simulink model "Problem3_ThreePhase_Inverter"  (R2025b)
settings: Solver=ode23t  StartTime=0.0  StopTime=0.1  MaxStep=1e-5  RelTol=1e-3
settings Model: Creator=Rashid  LastModifiedBy=Rashid

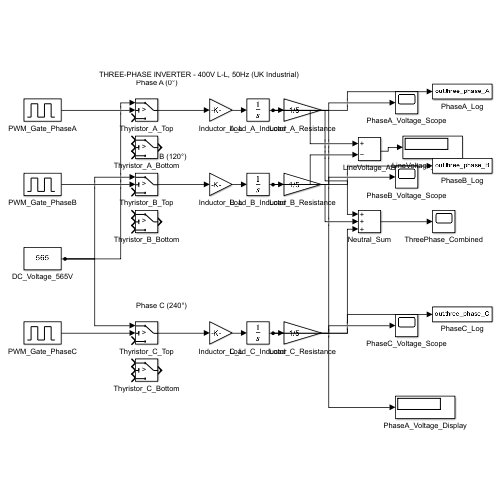
[thumbnail: Simulink's stored preview of the top-level diagram]
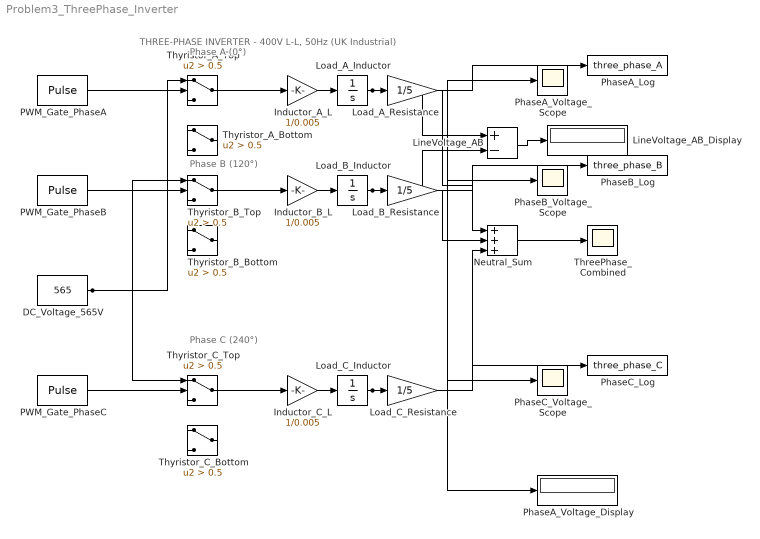
== system Problem3_ThreePhase_Inverter ==
  note: THREE-PHASE INVERTER - 400V L-L, 50Hz (UK Industrial)
  note: Phase A (0°)
  note: Phase B (120°)
  note: Phase C (240°)
  DC_Voltage_565V : Constant  Value=565
  Inductor_A_L : Gain  Gain=1/0.005
  Inductor_B_L : Gain  Gain=1/0.005
  Inductor_C_L : Gain  Gain=1/0.005
  LineVoltage_AB : Sum  Inputs=+-
  LineVoltage_AB_Display : Display
  Load_A_Inductor : Integrator
  Load_A_Resistance : Gain  Gain=1/5
  Load_B_Inductor : Integrator
  Load_B_Resistance : Gain  Gain=1/5
  Load_C_Inductor : Integrator
  Load_C_Resistance : Gain  Gain=1/5
  Neutral_Sum : Sum  Inputs=+++
  PWM_Gate_PhaseA : DiscretePulseGenerator  PulseType=Time based  Period=0.02  PulseWidth=33.3
  PWM_Gate_PhaseB : DiscretePulseGenerator  PulseType=Time based  Period=0.02  PulseWidth=33.3  PhaseDelay=0.00667
  PWM_Gate_PhaseC : DiscretePulseGenerator  PulseType=Time based  Period=0.02  PulseWidth=33.3  PhaseDelay=0.01333
  PhaseA_Log : ToWorkspace  VariableName=three_phase_A  SaveFormat=Timeseries  SampleTime=-1
  PhaseA_Voltage_Display : Display
  PhaseA_Voltage_Scope : Scope
  PhaseB_Log : ToWorkspace  VariableName=three_phase_B  SaveFormat=Timeseries  SampleTime=-1
  PhaseB_Voltage_Scope : Scope
  PhaseC_Log : ToWorkspace  VariableName=three_phase_C  SaveFormat=Timeseries  SampleTime=-1
  PhaseC_Voltage_Scope : Scope
  ThreePhase_Combined : Scope
  Thyristor_A_Bottom : Switch  Criteria=u2 > Threshold  Threshold=0.5  SaturateOnIntegerOverflow=off  InputSameDT=off
  Thyristor_A_Top : Switch  Criteria=u2 > Threshold  Threshold=0.5  SaturateOnIntegerOverflow=off  InputSameDT=off
  Thyristor_B_Bottom : Switch  Criteria=u2 > Threshold  Threshold=0.5  SaturateOnIntegerOverflow=off  InputSameDT=off
  Thyristor_B_Top : Switch  Criteria=u2 > Threshold  Threshold=0.5  SaturateOnIntegerOverflow=off  InputSameDT=off
  Thyristor_C_Bottom : Switch  Criteria=u2 > Threshold  Threshold=0.5  SaturateOnIntegerOverflow=off  InputSameDT=off
  Thyristor_C_Top : Switch  Criteria=u2 > Threshold  Threshold=0.5  SaturateOnIntegerOverflow=off  InputSameDT=off
  wires:
  PWM_Gate_PhaseA/1 -> Thyristor_A_Top/2
  DC_Voltage_565V/1 -> Thyristor_A_Top/1, Thyristor_B_Top/1, Thyristor_C_Top/1
  Thyristor_A_Top/1 -> Inductor_A_L/1
  Inductor_A_L/1 -> Load_A_Inductor/1
  Load_A_Inductor/1 -> Load_A_Resistance/1, PhaseA_Voltage_Scope/1, PhaseA_Log/1, LineVoltage_AB/1, PhaseA_Voltage_Display/1
  Load_A_Resistance/1 -> Neutral_Sum/1
  PWM_Gate_PhaseB/1 -> Thyristor_B_Top/2
  Thyristor_B_Top/1 -> Inductor_B_L/1
  Inductor_B_L/1 -> Load_B_Inductor/1
  Load_B_Inductor/1 -> Load_B_Resistance/1, PhaseB_Voltage_Scope/1, PhaseB_Log/1, LineVoltage_AB/2
  Load_B_Resistance/1 -> Neutral_Sum/2
  PWM_Gate_PhaseC/1 -> Thyristor_C_Top/2
  Thyristor_C_Top/1 -> Inductor_C_L/1
  Inductor_C_L/1 -> Load_C_Inductor/1
  Load_C_Inductor/1 -> Load_C_Resistance/1, PhaseC_Voltage_Scope/1, PhaseC_Log/1
  Load_C_Resistance/1 -> Neutral_Sum/3
  LineVoltage_AB/1 -> LineVoltage_AB_Display/1
  Neutral_Sum/1 -> ThreePhase_Combined/1
